simulink model "lookupTable"  (R2020a)
settings: Solver=VariableStepAuto  StartTime=0.0  StopTime=10.0  RelTol=1e-3
libraries: simulink x1
settings Model: Creator=royde  LastModifiedBy=royde

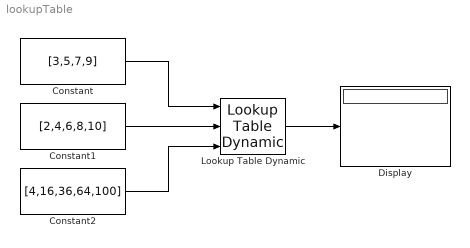
== system lookupTable ==
  Constant : Constant  Value=[3,5,7,9]
  Constant1 : Constant  Value=[2,4,6,8,10]
  Constant2 : Constant  Value=[4,16,36,64,100]
  Display : Display
  Lookup Table Dynamic : simulink/Lookup Tables/Lookup Table Dynamic  LookUpMeth=Interpolation-Use End Values  OutDataType=fixdt('double')  OutScaling=2^-10  OutputDataTypeScalingMode=Specify via dialog  OutDataTypeStr=double  DoSatur=off
  wires:
  Constant1/1 -> Lookup Table Dynamic/2
  Constant2/1 -> Lookup Table Dynamic/3
  Constant/1 -> Lookup Table Dynamic/1
  Lookup Table Dynamic/1 -> Display/1
